simulink model "cbf"  (R2023b)
settings: Solver=FixedStepAuto  StartTime=0.0  StopTime=inf  FixedStep=0.05  RelTol=1e-3
undefined symbols (not defined in the file): Angular, Linear
libraries: robotlib x19, dspstat3 x3
settings Model: Creator=ivory  LastModifiedBy=vanderbilt
settings SolverCC: AlgebraicLoopSolver=TrustRegion
settings OptimizationCC: EnhancedBackFolding=on  PassReuseOutputArgsAs=Individual arguments  ZeroExternalMemoryAtStartup=off  ZeroInternalMemoryAtStartup=off  MaxStackSize=64  OptimizeBlockOrder=speed  DifferentSizesBufferReuse=on  OptimizationCustomize=off  EfficientTunableParamExpr=on
settings DebuggingCC: ParameterTunabilityLossMsg=error  UnconnectedInputMsg=warning  UnconnectedOutputMsg=warning  UnconnectedLineMsg=warning
settings HardwareCC: ProdBitPerPointer=32  ProdBitPerSizeT=32  ProdBitPerPtrDiffT=32  ProdLargestAtomicFloat=None  ProdIntDivRoundTo=Undefined  ProdEndianess=Unspecified  ProdWordSize=32  ProdHWDeviceType=Generic->Unspecified (assume 32-bit Generic)
settings ModelReferenceCC: EnableRefExpFcnMdlSchedulingChecks=on
settings SFSimCC: MATLABDynamicMemAlloc=off  SimTargetLang=C++
settings RTWCC: Description=Embedded Coder  SystemTargetFile=ert.tlc  HardwareBoard=Robot Operating System (ROS)  TLCOptions="-aInlineSetEventsForThisBaseRateFcn=TLC_FALSE -aSuppressMultiTaskScheduler=TLC_FALSE  -aRateBasedStepFcn=0"  GenCodeOnly=on  TemplateMakefile=ert_default_tmf  GenerateReport=on  Toolchain=Catkin  IncludeHyperlinkInReport=on  LaunchReport=on  TargetLang=C++  GenerateTraceInfo=on  GenerateTraceReport=on  GenerateTraceReportSl=on  GenerateTraceReportSf=on  GenerateTraceReportEml=on  DLArmComputeVersion=19.05
settings CodeAppCC: ForceParamTrailComments=on  IgnoreCustomStorageClasses=off  OperatorAnnotations=on  SimulinkDataObjDesc=on  SFDataObjDesc=on  InsertBlockDesc=on
settings ERTTargetCC: SupportContinuousTime=on  SupportVariableSizeSignals=on

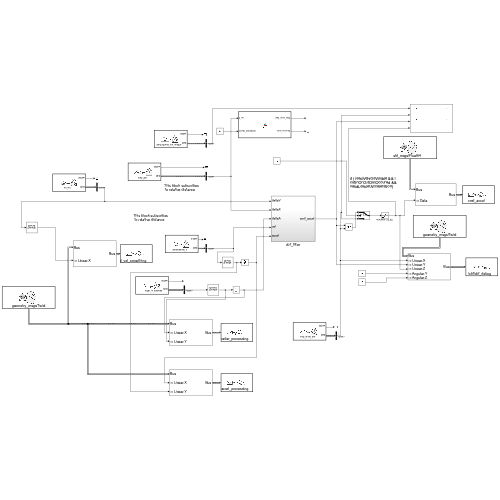
[thumbnail: Simulink's stored preview of the top-level diagram]
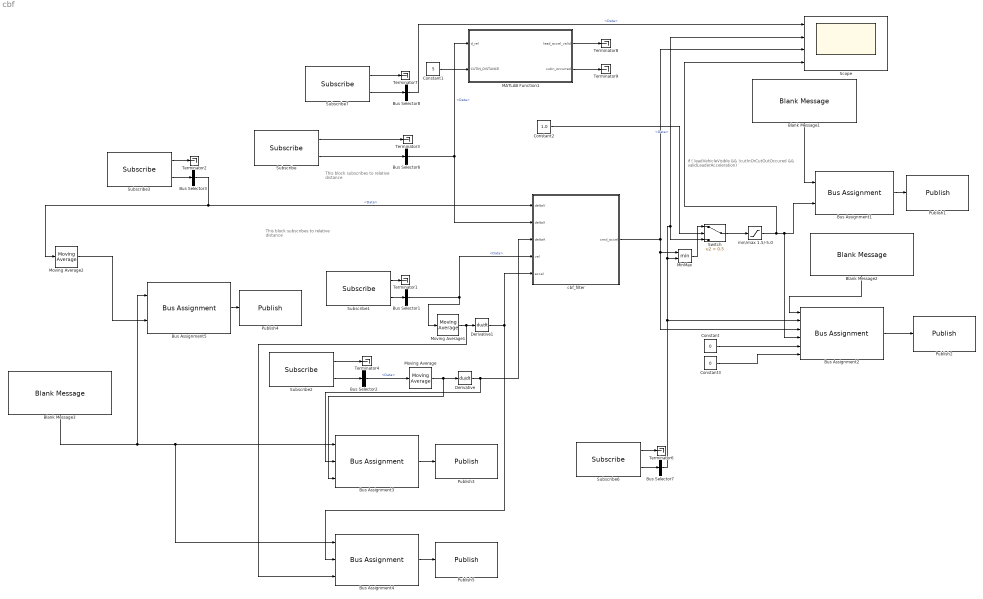
== system cbf ==
  note: if ( leadVehicleVisible && !cutInOrCutOutOccured && validLeaderAcceleration)
  note: This block subscribes
      | to relative distance
  note: This block subscribes
      | to relative distance
  Blank Message1 : robotlib/Blank Message  messageClass=Message  entityType=std_msgs/Float64  messageType=std_msgs/Float64  SampleTime=inf  legacyBusStruct=off
  Blank Message2 : robotlib/Blank Message  messageClass=Message  entityType=geometry_msgs/Twist  messageType=geometry_msgs/Twist  SampleTime=inf  legacyBusStruct=off
  Blank Message3 : robotlib/Blank Message  messageClass=Message  entityType=geometry_msgs/Twist  messageType=geometry_msgs/Twist  SampleTime=inf  legacyBusStruct=off
  Bus Assignment1 : BusAssignment  AssignedSignals=Data
  Bus Assignment2 : BusAssignment  AssignedSignals=Linear.X,Linear.Y,Linear.Z,Angular.Y,Angular.Z
  Bus Assignment3 : BusAssignment  AssignedSignals=Linear.X,Linear.Y
  Bus Assignment4 : BusAssignment  AssignedSignals=Linear.X,Linear.Y
  Bus Assignment5 : BusAssignment  AssignedSignals=Linear.X
  Bus Selector{1..3,6..8} (6 alike) : BusSelector  OutputSignals=Data
  Constant : Constant  Value=0
  Constant1 : Constant  Value=5
  Constant2 : Constant  Value=1.0
  Constant3 : Constant  Value=0
  Derivative : Derivative
  Derivative1 : Derivative
  MATLAB Function1 : MATLAB Function  TreatAsAtomicUnit=on
  MinMax : MinMax  Inputs=2
  Moving Average : dspstat3/Moving Average  Method=Sliding window  ForgettingFactorPort=off  SpecifyWindowLength=on  WindowLength=4  OverlapLength=3  AllowArbitraryInputLength=off  ForgettingFactor=0.9  SimulateUsing=Code generation
  Moving Average1 : dspstat3/Moving Average  Method=Sliding window  ForgettingFactorPort=off  SpecifyWindowLength=on  WindowLength=4  OverlapLength=3  AllowArbitraryInputLength=off  ForgettingFactor=0.9  SimulateUsing=Code generation
  Moving Average2 : dspstat3/Moving Average  Method=Sliding window  ForgettingFactorPort=off  SpecifyWindowLength=on  WindowLength=25  OverlapLength=24  AllowArbitraryInputLength=off  ForgettingFactor=0.9  SimulateUsing=Code generation
  Publish1 : robotlib/Publish  topicSource=Specify your own  topic=cmd_accel  messageType=std_msgs/Float64  legacyBusStruct=off  messageQueueLength=1
  Publish2 : robotlib/Publish  topicSource=Specify your own  topic=/cbf/cbf_debug  messageType=geometry_msgs/Twist  legacyBusStruct=off  messageQueueLength=1
  Publish3 : robotlib/Publish  topicSource=Specify your own  topic=radar_processing  messageType=geometry_msgs/Twist  legacyBusStruct=off  messageQueueLength=1
  Publish4 : robotlib/Publish  topicSource=Specify your own  topic=rel_vel_smoothing  messageType=geometry_msgs/Twist  legacyBusStruct=off  messageQueueLength=1
  Publish5 : robotlib/Publish  topicSource=Specify your own  topic=accel_processing  messageType=geometry_msgs/Twist  legacyBusStruct=off  messageQueueLength=1
  Scope : Scope  NumInputPorts=4
  Subscribe : robotlib/Subscribe  topicSource=Specify your own  topic=lead_dist  messageType=std_msgs/Float64  SampleTime=-1  legacyBusStruct=off  messageQueueLength=1
  Subscribe1 : robotlib/Subscribe  topicSource=Specify your own  topic=/car/state/vel_x  messageType=std_msgs/Float64  SampleTime=-1  legacyBusStruct=off  messageQueueLength=1
  Subscribe2 : robotlib/Subscribe  topicSource=Specify your own  topic=radar_rv_estimate  messageType=std_msgs/Float64  SampleTime=-1  legacyBusStruct=off  messageQueueLength=1
  Subscribe3 : robotlib/Subscribe  topicSource=Specify your own  topic=rel_vel  messageType=std_msgs/Float64  SampleTime=-1  legacyBusStruct=off  messageQueueLength=1
  Subscribe6 : robotlib/Subscribe  topicSource=Specify your own  topic=cmd_accel_pre  messageType=std_msgs/Float64  SampleTime=-1  legacyBusStruct=off  messageQueueLength=1
  Subscribe7 : robotlib/Subscribe  topicSource=Specify your own  topic=/car/hud/mini_car_enable  messageType=std_msgs/Bool  SampleTime=-1  legacyBusStruct=off  messageQueueLength=1
  Switch : Switch  Criteria=u2 > Threshold  Threshold=0.5  SaturateOnIntegerOverflow=off  InputSameDT=off
  Terminator{1..4,6..9} (8 alike) : Terminator
  cbf_filter : Subsystem
  min/max 1.5/-5.0 : Saturate  UpperLimit=1.5  LowerLimit=-5.0
  wires:
  MATLAB Function1/1(lead_accel_valid) -> Terminator8/1
  MinMax/1 -> Switch/1
  Bus Selector8/1 -> Scope/1  "<Data>"
  Subscribe7/2 -> Bus Selector8/1
  Subscribe2/1 -> Terminator4/1
  Subscribe1/1 -> Terminator1/1
  Bus Assignment1/1 -> Publish1/1
  Bus Selector7/1 -> Bus Assignment2/2, MinMax/2, Switch/3, Scope/2  "<Data>"
  Subscribe2/2 -> Bus Selector2/1
  cbf_filter/1(cmd_accel) -> Scope/3, Bus Assignment2/3, MinMax/1
  Bus Selector6/1 -> MATLAB Function1/1(d_rel), cbf_filter/2(deltaX)  "<Data>"
  Bus Assignment2/1 -> Publish2/1
  Subscribe7/1 -> Terminator7/1
  Subscribe/1 -> Terminator3/1
  Constant1/1 -> MATLAB Function1/2(CUTIN_DISTANCE)
  Switch/1 -> min/max 1.5/-5.0/1
  Bus Selector2/1 -> Moving Average/1  "<Data>"
  Subscribe6/1 -> Terminator6/1
  Blank Message1/1 -> Bus Assignment1/1
  min/max 1.5/-5.0/1 -> Scope/4, Bus Assignment2/4, Bus Assignment1/2
  Subscribe1/2 -> Bus Selector1/1
  MATLAB Function1/2(cutin_occurred) -> Terminator9/1
  Bus Selector1/1 -> Moving Average1/1, cbf_filter/4(vel)  "<Data>"
  Subscribe/2 -> Bus Selector6/1
  Constant2/1 -> Switch/2
  Blank Message2/1 -> Bus Assignment2/1
  Subscribe6/2 -> Bus Selector7/1
  Derivative1/1 -> Bus Assignment4/2, cbf_filter/5(accel)
  Constant/1 -> Bus Assignment2/5
  Constant3/1 -> Bus Assignment2/6
  Moving Average/1 -> Bus Assignment3/3, Derivative/1
  Moving Average1/1 -> Bus Assignment4/3, Derivative1/1
  Derivative/1 -> cbf_filter/3(deltaA), Bus Assignment3/2
  Blank Message3/1 -> Bus Assignment4/1, Bus Assignment3/1, Bus Assignment5/1
  Bus Assignment3/1 -> Publish3/1
  Bus Assignment4/1 -> Publish5/1
  Subscribe3/1 -> Terminator2/1
  Subscribe3/2 -> Bus Selector3/1
  Bus Selector3/1 -> Moving Average2/1, cbf_filter/1(deltaV)  "<Data>"
  Bus Assignment5/1 -> Publish4/1
  Moving Average2/1 -> Bus Assignment5/2

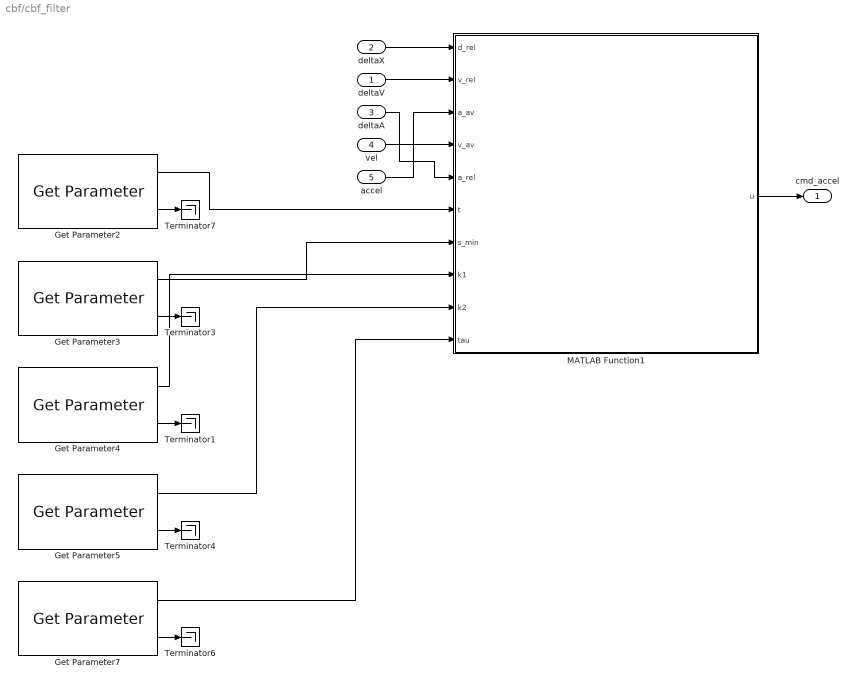
== system cbf/cbf_filter ==
  deltaV : Inport
  deltaX : Inport  Port=2
  deltaA : Inport  Port=3
  vel : Inport  Port=4
  accel : Inport  Port=5
  Get Parameter2 : robotlib/Get Parameter  ParameterSource=Specify your own  ParameterName=timegap  ParameterType=double  ParameterMaxArrayLength=16  ParameterInitialValue=2.0  SampleTime=-1  ShowErrorCodeOutput=on  ModelName=cbf  BlockId=ParamGet_cbf_567
  Get Parameter3 : robotlib/Get Parameter  ParameterSource=Specify your own  ParameterName=s_min  ParameterType=double  ParameterMaxArrayLength=16  ParameterInitialValue=7.0  SampleTime=-1  ShowErrorCodeOutput=on  ModelName=cbf  BlockId=ParamGet_cbf_568
  Get Parameter4 : robotlib/Get Parameter  ParameterSource=Specify your own  ParameterName=k1  ParameterType=double  ParameterMaxArrayLength=16  ParameterInitialValue=0.5  SampleTime=-1  ShowErrorCodeOutput=on  ModelName=cbf  BlockId=ParamGet_cbf_569
  Get Parameter5 : robotlib/Get Parameter  ParameterSource=Specify your own  ParameterName=k2  ParameterType=double  ParameterMaxArrayLength=16  ParameterInitialValue=0.5  SampleTime=-1  ShowErrorCodeOutput=on  ModelName=cbf  BlockId=ParamGet_cbf_570
  Get Parameter7 : robotlib/Get Parameter  ParameterSource=Specify your own  ParameterName=tau  ParameterType=double  ParameterMaxArrayLength=16  ParameterInitialValue=1.5  SampleTime=-1  ShowErrorCodeOutput=on  ModelName=cbf  BlockId=ParamGet_cbf_595
  MATLAB Function1 : MATLAB Function  TreatAsAtomicUnit=on
  Terminator{1,3..4,6..7} (5 alike) : Terminator
  cmd_accel : Outport
  wires:
  Get Parameter4/1 -> MATLAB Function1/8(k1)
  Get Parameter4/2 -> Terminator1/1
  Get Parameter2/1 -> MATLAB Function1/6(t)
  Get Parameter2/2 -> Terminator7/1
  Get Parameter3/2 -> Terminator3/1
  Get Parameter3/1 -> MATLAB Function1/7(s_min)
  MATLAB Function1/1(u) -> cmd_accel/1
  vel/1 -> MATLAB Function1/4(v_av)
  deltaV/1 -> MATLAB Function1/2(v_rel)
  deltaX/1 -> MATLAB Function1/1(d_rel)
  Get Parameter5/2 -> Terminator4/1
  Get Parameter5/1 -> MATLAB Function1/9(k2)
  deltaA/1 -> MATLAB Function1/5(a_rel)
  accel/1 -> MATLAB Function1/3(a_av)
  Get Parameter7/2 -> Terminator6/1
  Get Parameter7/1 -> MATLAB Function1/10(tau)

== matlab function cbf/cbf_filter/MATLAB Function1 ==
  data: u output; d_rel input; v_rel input; a_av input; v_av input; a_rel input; t input; s_min input; k1 input; k2 input; tau input
function u = fcn(d_rel,v_rel,a_av, v_av, a_rel, t,s_min,k1,k2,tau)
%% calculates cbf acceleration given a model with first-order lag on accel:

h = (d_rel - t*v_av - s_min);

dh_dt = (v_rel - t*a_av);

u = (tau/t)*(a_rel + (t/tau)*a_av + (k1+k2)*(dh_dt) + (k1*k2)*h);

== matlab function cbf/MATLAB Function1 ==
  data: lead_accel_valid output; d_rel input; CUTIN_DISTANCE input; cutin_occurred output
function [lead_accel_valid, cutin_occurred]= fcn(d_rel,CUTIN_DISTANCE)
%#codegen

persistent relative_distance_prev;
if isempty(relative_distance_prev)
    relative_distance_prev=d_rel;
end

cutin_occurred = 1;
lead_accel_valid=1;

if( abs( relative_distance_prev - d_rel ) > CUTIN_DISTANCE )
    cutin_occurred = 1;
else
    cutin_occurred = 0;
end

relative_distance_prev = d_rel;
